simulink model "video"  (Simulink 7.2)
settings: Solver=ode45  StartTime=0.0  StopTime=3  RelTol=1e-3
undefined symbols (not defined in the file or in its folder): gray, none, Rec, SDTV, videoinput
libraries: vipsnks x2, vipconversions x1, vipanalysis x1, imaqlib x1
settings Model: Creator=Gus  LastModifiedBy=Gus
settings SimEventsCC: propLogEventsScheduled=0  propLogEventsExecuted=0  propLogDepartureEvents=0  propDisplayEventCalendar=0  propDiagAttribOutput=1  propDiagFcnCallOutput=1  propDiagStatOutput=0

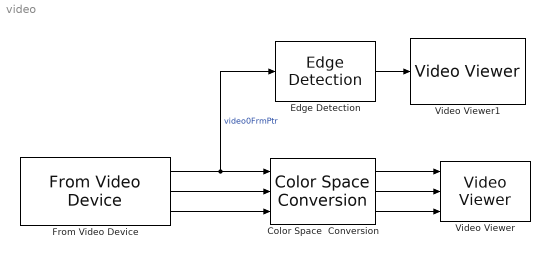
== system video ==
  Color Space  Conversion : vipconversions/Color Space  Conversion  conversion=Obsolete  conversionActive=Y'CbCr to R'G'B'  wp_str=D65  rec=Rec. 601 (SDTV)  sys=1125/60/2:1  imagePorts=Separate color signals
  Edge Detection : vipanalysis/Edge Detection  DialogController=vipDDGCreate  DialogControllerArgs=DataTag0  method=Sobel  outputType=Binary image  userDefinedThreshold=off  thresholdSource=Input port  threshold=20  thresholdTuning=3  edgeThinning=off  threshold_canny=[0.25 0.60]  autoPercent=70  sigma=1  prodOutputMode=Binary point scaling  prodOutputWordLength=32  prodOutputFracLength=8  roundingMode=Floor  overflowMode=off
  From Video Device : imaqlib/From Video Device  DialogController=imaqcreatedialog  DialogControllerArgs=DataTag2  DeviceMenu=winvideo 1 (Dispositivo de vídeo USB)  Device=winvideo 1 (Dispositivo de vídeo USB)  ObjConstructor=videoinput('winvideo', 1)  VideoFormatMenu=YUY2_320x240  VideoFormat=YUY2_320x240  VideoSource=input1  ROIPosition=[0 0 240 320]  EnableHWTrigger=off  TriggerConfiguration=none/none  SampleTime=1/30  OutputPortsMode=Separate color signals  DataType=single  CanDoHWTrigger=no  ReturnedColorSpace=YCbCr  BlockHandle=1871.002  ROIWidth=320  ROIHeight=240
  Video Viewer : vipsnks/Video Viewer  DialogController=vipDDGCreate  DialogControllerArgs=DataTag3  inputType=Obsolete7b  imagePorts=Separate color signals  useColorMap=off  colormapValue=gray(256)  specRange=off  minInputVal=0  maxInputVal=255  FigPos=[630 593 640 480]  AxisZoom=on  trueSizedOnce=on
  Video Viewer1 : vipsnks/Video Viewer  DialogController=vipDDGCreate  DialogControllerArgs=DataTag4  inputType=Obsolete7b  imagePorts=One multidimensional signal  useColorMap=off  colormapValue=gray(256)  specRange=off  minInputVal=0  maxInputVal=255  FigPos=[630 593 640 480]  AxisZoom=on  trueSizedOnce=on
  wires:
  From Video Device/1 -> Edge Detection/1, Color Space  Conversion/1  "video0FrmPtr"
  Edge Detection/1 -> Video Viewer1/1
  Color Space  Conversion/1 -> Video Viewer/1
  Color Space  Conversion/2 -> Video Viewer/2
  Color Space  Conversion/3 -> Video Viewer/3
  From Video Device/2 -> Color Space  Conversion/2
  From Video Device/3 -> Color Space  Conversion/3
